simulink subsystem "HIL"  (R2024a)
settings: Solver=VariableStepAuto  StartTime=0.0  StopTime=10.0  RelTol=1e-3
values from neighbouring files (symbols this model uses):
  Hil = 100.0    [ModelDD.sldd]
  Sim : value not decoded    [ModelDD.sldd]
undefined symbols (not defined in the file or in its folder): D1, Delta, DiscIntNeverNeededParam
libraries: simulink x60, spsSeriesRLCBranchLib x18, spsControlledVoltageSourceLib x15, spsThreePhaseVIMeasurementLib x9, spsGroundLib x8, hdlsllib x6, spsMosfetLib x6, spsabctodq0Lib x5, spsDCVoltageSourceLib x3, spsPower3phInstantaneousLib x3, spsVoltageMeasurementLib x3, spspowerguiLib x3
(part 3 of 3)

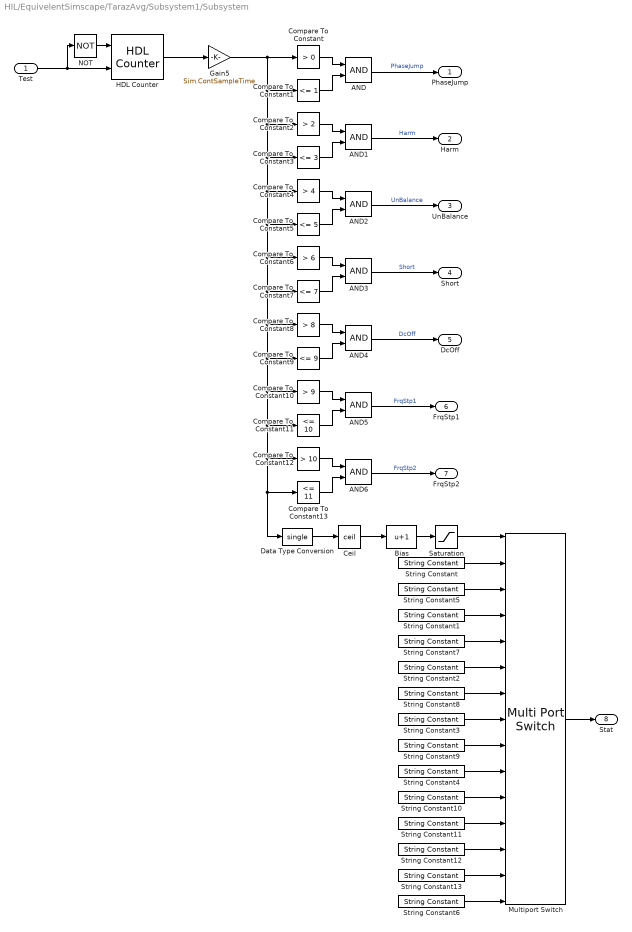
== system HIL/EquivelentSimscape/TarazAvg/Subsystem1/Subsystem ==
  Test : Inport
  AND{,1..6} (7 alike) : Logic  AllPortsSameDT=off  OutDataTypeStr=boolean
  Bias : Bias  Bias=1  SaturateOnIntegerOverflow=off
  Ceil : Rounding  Operator=ceil
  Compare To Constant : simulink/Logic and Bit Operations/Compare To Constant  relop=>  const=0  OutDataTypeStr=boolean
  Compare To Constant1 : simulink/Logic and Bit Operations/Compare To Constant  relop=<=  const=1  OutDataTypeStr=boolean
  Compare To Constant10 : simulink/Logic and Bit Operations/Compare To Constant  relop=>  const=9  OutDataTypeStr=boolean
  Compare To Constant11 : simulink/Logic and Bit Operations/Compare To Constant  relop=<=  const=10  OutDataTypeStr=boolean
  Compare To Constant12 : simulink/Logic and Bit Operations/Compare To Constant  relop=>  const=10  OutDataTypeStr=boolean
  Compare To Constant13 : simulink/Logic and Bit Operations/Compare To Constant  relop=<=  const=11  OutDataTypeStr=boolean
  Compare To Constant2 : simulink/Logic and Bit Operations/Compare To Constant  relop=>  const=2  OutDataTypeStr=boolean
  Compare To Constant3 : simulink/Logic and Bit Operations/Compare To Constant  relop=<=  const=3  OutDataTypeStr=boolean
  Compare To Constant4 : simulink/Logic and Bit Operations/Compare To Constant  relop=>  const=4  OutDataTypeStr=boolean
  Compare To Constant5 : simulink/Logic and Bit Operations/Compare To Constant  relop=<=  const=5  OutDataTypeStr=boolean
  Compare To Constant6 : simulink/Logic and Bit Operations/Compare To Constant  relop=>  const=6  OutDataTypeStr=boolean
  Compare To Constant7 : simulink/Logic and Bit Operations/Compare To Constant  relop=<=  const=7  OutDataTypeStr=boolean
  Compare To Constant8 : simulink/Logic and Bit Operations/Compare To Constant  relop=>  const=8  OutDataTypeStr=boolean
  Compare To Constant9 : simulink/Logic and Bit Operations/Compare To Constant  relop=<=  const=9  OutDataTypeStr=boolean
  Data Type Conversion : DataTypeConversion  OutDataTypeStr=single  SaturateOnIntegerOverflow=off  RndMeth=Floor
  Gain5 : Gain  Gain=Sim.ContSampleTime  ParamDataTypeStr=double  OutDataTypeStr=double
  HDL Counter : hdlsllib/Sources/HDL Counter  CountType=Free running  CountInit=0  CountStep=1  CountMax=25  CountFromType=Initial value  CountFrom=0  CountResetPort=on  CountLoadPort=off  CountEnbPort=on  CountDirPort=off  CountHitOutputPort=off  CountDataType=Unsigned  CountWordLen=32  CountFracLen=0  CountSampTime=1
  Multiport Switch : MultiPortSwitch  Inputs=14  SaturateOnIntegerOverflow=off  InputSameDT=off
  NOT : Logic  Operator=NOT  AllPortsSameDT=off  OutDataTypeStr=boolean
  Saturation : Saturate  UpperLimit=14  LowerLimit=0
  String Constant{,1..4,6,11} (7 alike) : StringConstant  String="\"Normal\""
  String Constant10 : StringConstant  String="\"DC Offset\""
  String Constant12 : StringConstant  String="\"Freq Stp 1\""
  String Constant13 : StringConstant  String="\"Freq Stp 2\""
  String Constant5 : StringConstant  String="\"Phase Jump\""
  String Constant7 : StringConstant  String="\"Harm\""
  String Constant8 : StringConstant  String="\"Unbalance\""
  String Constant9 : StringConstant  String="\"Short\""
  PhaseJump : Outport
  Harm : Outport  Port=2
  UnBalance : Outport  Port=3
  Short : Outport  Port=4
  DcOff : Outport  Port=5
  FrqStp1 : Outport  Port=6
  FrqStp2 : Outport  Port=7
  Stat : Outport  Port=8
  wires:
  Bias/1 -> Saturation/1
  Data Type Conversion/1 -> Ceil/1
  Multiport Switch/1 -> Stat/1
  Saturation/1 -> Multiport Switch/1
  Ceil/1 -> Bias/1
  String Constant13/1 -> Multiport Switch/14
  String Constant12/1 -> Multiport Switch/13
  String Constant11/1 -> Multiport Switch/12
  String Constant10/1 -> Multiport Switch/11
  String Constant9/1 -> Multiport Switch/9
  String Constant8/1 -> Multiport Switch/7
  String Constant7/1 -> Multiport Switch/5
  String Constant5/1 -> Multiport Switch/3
  String Constant6/1 -> Multiport Switch/15
  String Constant4/1 -> Multiport Switch/10
  String Constant3/1 -> Multiport Switch/8
  String Constant2/1 -> Multiport Switch/6
  String Constant1/1 -> Multiport Switch/4
  String Constant/1 -> Multiport Switch/2
  NOT/1 -> HDL Counter/1
  Compare To Constant13/1 -> AND6/2
  Compare To Constant12/1 -> AND6/1
  AND6/1 -> FrqStp2/1  "FrqStp2"
  AND5/1 -> FrqStp1/1  "FrqStp1"
  Compare To Constant10/1 -> AND5/1
  Compare To Constant11/1 -> AND5/2
  AND/1 -> PhaseJump/1  "PhaseJump"
  Test/1 -> HDL Counter/2, NOT/1
  AND2/1 -> UnBalance/1  "UnBalance"
  AND3/1 -> Short/1  "Short"
  HDL Counter/1 -> Gain5/1
  Compare To Constant5/1 -> AND2/2
  Compare To Constant/1 -> AND/1
  Compare To Constant9/1 -> AND4/2
  Compare To Constant2/1 -> AND1/1
  Compare To Constant8/1 -> AND4/1
  Compare To Constant3/1 -> AND1/2
  AND4/1 -> DcOff/1  "DcOff"
  Compare To Constant1/1 -> AND/2
  Compare To Constant7/1 -> AND3/2
  Compare To Constant6/1 -> AND3/1
  Gain5/1 -> Compare To Constant/1, Compare To Constant1/1, Compare To Constant3/1, Compare To Constant5/1, Compare To Constant7/1, Compare To Constant8/1, Compare To Constant9/1, Compare To Constant13/1, Data Type Conversion/1, Compare To Constant12/1, Compare To Constant11/1, Compare To Constant10/1, Compare To Constant6/1, Compare To Constant4/1, Compare To Constant2/1
  AND1/1 -> Harm/1  "Harm"
  Compare To Constant4/1 -> AND2/1

== system HIL/EquivelentSimscape/TarazAvg/Subsystem1/WrappedIntegrator ==
  w : Inport
  Constant1 : Constant  Value=2*pi
  Discrete-Time Integrator1 : DiscreteIntegrator  gainval=single(1)  ExternalReset=rising  InitialConditionSource=external  SampleTime=-1  ShowStatePort=on  ICPrevOutput=DiscIntNeverNeededParam  ICPrevScaledInput=DiscIntNeverNeededParam
  GreaterThan : RelationalOperator  Operator=~=  OutDataTypeStr=boolean  RndMeth=Simplest  InputSameDT=off
  Mod : Math  Operator=mod
  wt : Outport
  wires:
  GreaterThan/1 -> Discrete-Time Integrator1/2
  Discrete-Time Integrator1/1 -> wt/1  "wt"
  w/1 -> Discrete-Time Integrator1/1
  Discrete-Time Integrator1/State -> Mod/1, GreaterThan/1
  Mod/1 -> GreaterThan/2, Discrete-Time Integrator1/3
  Constant1/1 -> Mod/2

== system HIL/PWM/PWM/PWM Generator/Carrier ==
  Enable : Inport  OutDataTypeStr=boolean  PortDimensions=1
  PWM Period : Inport  Port=2  OutDataTypeStr=uint32  PortDimensions=1
  Abs : Abs  OutDataTypeStr=uint32  SaturateOnIntegerOverflow=off
  Bias : Bias  Bias=-1  SaturateOnIntegerOverflow=off
  Data Type Conversion : DataTypeConversion  OutDataTypeStr=int32  SaturateOnIntegerOverflow=off  RndMeth=Floor
  HDL Counter : hdlsllib/Sources/HDL Counter  CountType=Free running  CountInit=0  CountStep=1  CountMax=25  CountFromType=Initial value  CountFrom=0  CountResetPort=on  CountLoadPort=off  CountEnbPort=on  CountDirPort=off  CountHitOutputPort=off  CountDataType=Unsigned  CountWordLen=32  CountFracLen=0  CountSampTime=1
  Minus : Sum  Inputs=+-  OutDataTypeStr=int32
  Multiply : Gain  Gain=2  OutDataTypeStr=uint32
  NOT : Logic  Operator=NOT  AllPortsSameDT=off  OutDataTypeStr=boolean
  OR : Logic  Operator=OR  AllPortsSameDT=off  OutDataTypeStr=boolean
  Relational Operator : RelationalOperator  OutDataTypeStr=boolean  InputSameDT=off
  Counter : Outport  VectorParamsAs1DForOutWhenUnconnected=off
  Trig : Outport  Port=2  VectorParamsAs1DForOutWhenUnconnected=off
  wires:
  Relational Operator/1 -> Trig/1, OR/1
  HDL Counter/1 -> Relational Operator/1, Minus/1
  Enable/1 -> NOT/1, HDL Counter/2
  PWM Period/1 -> Multiply/1, Minus/2
  Minus/1 -> Abs/1
  Abs/1 -> Counter/1  "Carrier_Cnt"
  Multiply/1 -> Data Type Conversion/1
  OR/1 -> HDL Counter/1
  NOT/1 -> OR/2
  Bias/1 -> Relational Operator/2
  Data Type Conversion/1 -> Bias/1
